simulink model "simplifiedTxTestbench"  (R2024a)
settings: Solver=FixedStepDiscrete  StartTime=0.0  StopTime=stopTime  RelTol=1e-3
values from neighbouring files (symbols this model uses):
  pWords = [pWords binl2str(pBitsRaw)]    [simplifiedTb.m]    (also in tx.m = [pWords binl2str(pBitsRaw{i})])
  reg0 = zeros(length(msgIn), 1)    [tx.m]
  reg1 = zeros(length(msgIn), 1)    [tx.m]
  reg2 = zeros(length(msgIn), 1)    [tx.m]
  reg3 = zeros(length(msgIn), 1)    [tx.m]
undefined symbols (not defined in the file or in its folder): fDAC, fPHY, fs
libraries: dspsrcs4 x3, HDL_ieee_8021513 x2, hdlsllib x1, whdlutilities x1
settings Model: DataTypeOverride=Off  SimulationMode=accelerator  Creator=cotti  LastModifiedBy=cotti
settings OptimizationCC: BlockReduction=off  ConditionallyExecuteInputs=off  DefaultParameterBehavior=Inlined  InheritOutputTypeSmallerThanSingle=on
settings DebuggingCC: ArtificialAlgebraicLoopMsg=error  SingleTaskRateTransMsg=error
settings HardwareCC: ProdBitPerPointer=32  ProdBitPerSizeT=32  ProdBitPerPtrDiffT=32  ProdLargestAtomicFloat=None  ProdIntDivRoundTo=Undefined  ProdEndianess=Unspecified  ProdWordSize=32  ProdHWDeviceType=ASIC/FPGA->ASIC/FPGA  TargetBitPerLong=64  TargetBitPerPointer=64  TargetBitPerSizeT=64  TargetBitPerPtrDiffT=64  TargetLongLongMode=on  TargetIntDivRoundTo=Zero  TargetEndianess=LittleEndian  TargetWordSize=64  TargetHWDeviceType=Custom Processor->MATLAB Host Computer  ProdEqTarget=off

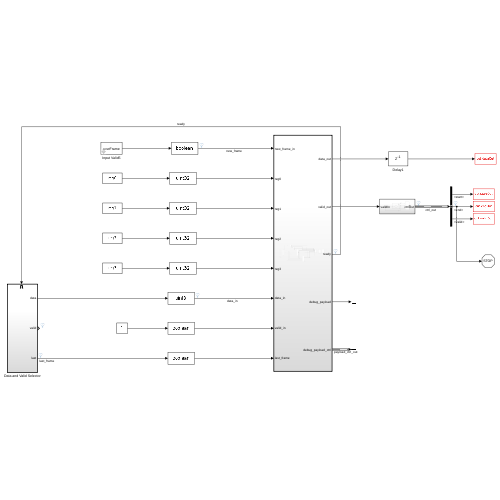
[thumbnail: Simulink's stored preview of the top-level diagram]
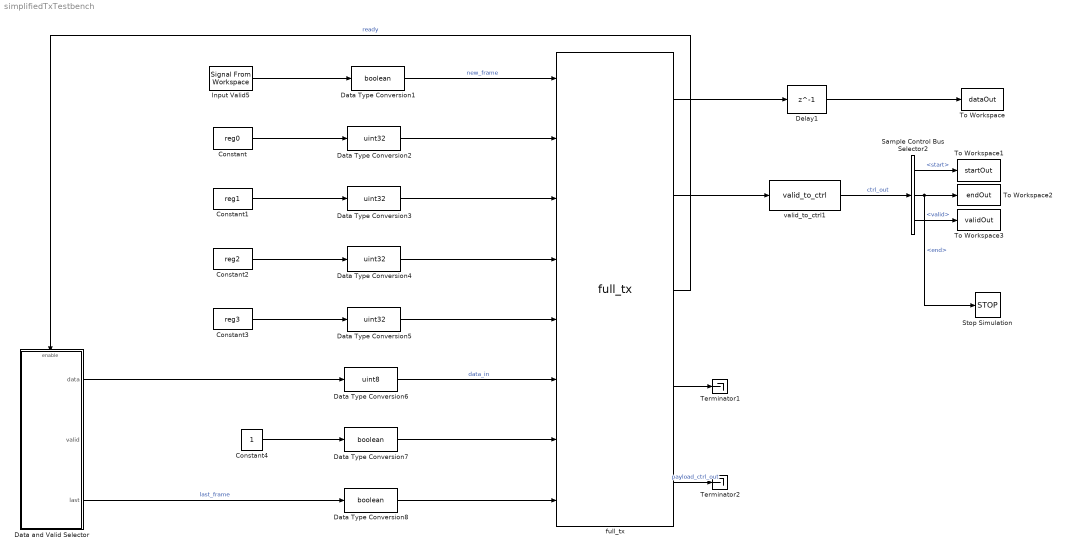
== system simplifiedTxTestbench ==
  Constant : Constant  Value=reg0  OutDataTypeStr=uint32  SampleTime=8/fs
  Constant1 : Constant  Value=reg1  OutDataTypeStr=uint32  SampleTime=8/fs
  Constant2 : Constant  Value=reg2  OutDataTypeStr=uint32  SampleTime=8/fs
  Constant3 : Constant  Value=reg3  OutDataTypeStr=uint32  SampleTime=8/fs
  Constant4 : Constant  SampleTime=-1
  Data Type Conversion1 : DataTypeConversion  OutDataTypeStr=boolean  SaturateOnIntegerOverflow=off  RndMeth=Floor
  Data Type Conversion{2..5} (4 alike) : DataTypeConversion  OutDataTypeStr=uint32  SaturateOnIntegerOverflow=off  RndMeth=Floor
  Data Type Conversion6 : DataTypeConversion  OutDataTypeStr=uint8  SaturateOnIntegerOverflow=off  RndMeth=Floor
  Data Type Conversion7 : DataTypeConversion  OutDataTypeStr=boolean  SaturateOnIntegerOverflow=off  RndMeth=Floor
  Data Type Conversion8 : DataTypeConversion  OutDataTypeStr=boolean  SaturateOnIntegerOverflow=off  RndMeth=Floor
  Data and Valid Selector : Subsystem  TreatAsAtomicUnit=on
  Delay1 : Delay  DelayLength=1  InitialCondition=0  UseCircularBuffer=on
  Input Valid5 : dspsrcs4/Signal From Workspace  X=newFrame  Ts=1/(fPHY/4)  nsamps=1  OutputAfterFinalValue=Setting to zero  ignoreOrWarnInputAndFrameLengths=off  OutputFrames=off
  Sample Control Bus Selector2 : whdlutilities/Sample Control Bus Selector  OutputSignals=start,end,valid
  Stop Simulation : Stop
  Terminator1 : Terminator
  Terminator2 : Terminator
  To Workspace : ToWorkspace  VariableName=dataOut  SampleTime=1/fDAC
      settings: Save2DSignal=2-D array (concatenate along first dimension)
  To Workspace1 : ToWorkspace  VariableName=startOut  SampleTime=1/fDAC
      settings: Save2DSignal=2-D array (concatenate along first dimension)
  To Workspace2 : ToWorkspace  VariableName=endOut  SampleTime=1/fDAC
      settings: Save2DSignal=2-D array (concatenate along first dimension)
  To Workspace3 : ToWorkspace  VariableName=validOut  SampleTime=1/fDAC
      settings: Save2DSignal=2-D array (concatenate along first dimension)
  full_tx : HDL_ieee_8021513/full_tx  SystemSampleTime=-1  VariantActivationTime=update diagram  AllowFlexibleInterface=on  Latency=0  AutoFrameSizeCalculation=off
      settings: SourceProductName=HDL IEEE 8021513
  valid_to_ctrl1 : HDL_ieee_8021513/valid_to_ctrl  SystemSampleTime=-1  VariantActivationTime=update diagram  AllowFlexibleInterface=on  Latency=0  AutoFrameSizeCalculation=off
      settings: SourceProductName=HDL IEEE 8021513
  wires:
  full_tx/3 -> Data and Valid Selector/Enable  "ready"
  Data Type Conversion1/1 -> full_tx/1  "new_frame"
  Data Type Conversion4/1 -> full_tx/4
  Constant2/1 -> Data Type Conversion4/1
  valid_to_ctrl1/1 -> Sample Control Bus Selector2/1  "ctrl_out"
  Data and Valid Selector/1(data) -> Data Type Conversion6/1
  Constant/1 -> Data Type Conversion2/1
  Data Type Conversion5/1 -> full_tx/5
  full_tx/2 -> valid_to_ctrl1/1
  Data and Valid Selector/3(last) -> Data Type Conversion8/1  "last_frame"
  full_tx/1 -> Delay1/1
  Data Type Conversion3/1 -> full_tx/3
  Delay1/1 -> To Workspace/1
  Constant1/1 -> Data Type Conversion3/1
  Sample Control Bus Selector2/3 -> To Workspace3/1  "<valid>"
  Constant3/1 -> Data Type Conversion5/1
  Input Valid5/1 -> Data Type Conversion1/1
  Data Type Conversion2/1 -> full_tx/2
  Sample Control Bus Selector2/1 -> To Workspace1/1  "<start>"
  Data Type Conversion6/1 -> full_tx/6  "data_in"
  Sample Control Bus Selector2/2 -> To Workspace2/1, Stop Simulation/1  "<end>"
  Data Type Conversion8/1 -> full_tx/8
  full_tx/4 -> Terminator1/1
  full_tx/5 -> Terminator2/1  "payload_ctrl_out"
  Constant4/1 -> Data Type Conversion7/1
  Data Type Conversion7/1 -> full_tx/7

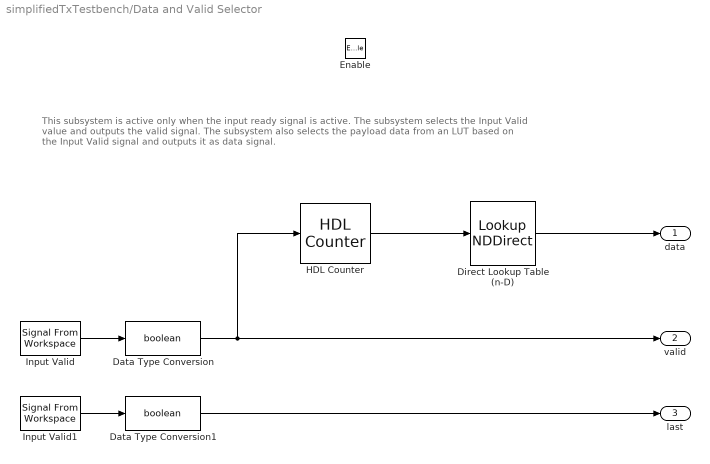
== system simplifiedTxTestbench/Data and Valid Selector ==
  note: This subsystem is active only when the input ready signal is active. The subsystem selects the Input Valid value and outputs the valid signal.
      | The subsystem also selects the payload data from an LUT based on the Input Valid signal and outputs it as data signal.
  Enable : EnablePort
  Data Type Conversion : DataTypeConversion  OutDataTypeStr=boolean  SaturateOnIntegerOverflow=off  RndMeth=Floor
  Data Type Conversion1 : DataTypeConversion  OutDataTypeStr=boolean  SaturateOnIntegerOverflow=off  RndMeth=Floor
  Direct Lookup Table (n-D) : LookupNDDirect  NumberOfTableDimensions=1  Table=uint8(pWords')  DiagnosticForOutOfRangeInput=Error  TableDataTypeStr=uint8
  HDL Counter : hdlsllib/Sources/HDL Counter  CountType=Count limited  CountInit=0  CountStep=1  CountMax=length(pWords) -1  CountFromType=Initial value  CountFrom=0  CountResetPort=off  CountLoadPort=off  CountEnbPort=on  CountDirPort=off  CountHitOutputPort=off  CountDataType=Unsigned  CountWordLen=nextpow2(length(pWords))  CountFracLen=0  CountSampTime=1
  Input Valid : dspsrcs4/Signal From Workspace  X=validIn  Ts=1/(fPHY/4)  nsamps=1  OutputAfterFinalValue=Setting to zero  ignoreOrWarnInputAndFrameLengths=off  OutputFrames=off
  Input Valid1 : dspsrcs4/Signal From Workspace  X=lastIn  Ts=1/(fPHY/4)  nsamps=1  OutputAfterFinalValue=Setting to zero  ignoreOrWarnInputAndFrameLengths=off  OutputFrames=off
  data : Outport  InitialOutput=0  VectorParamsAs1DForOutWhenUnconnected=off
  valid : Outport  Port=2  InitialOutput=0  VectorParamsAs1DForOutWhenUnconnected=off
  last : Outport  Port=3  VectorParamsAs1DForOutWhenUnconnected=off
  wires:
  HDL Counter/1 -> Direct Lookup Table (n-D)/1
  Direct Lookup Table (n-D)/1 -> data/1
  Input Valid/1 -> Data Type Conversion/1
  Data Type Conversion/1 -> valid/1, HDL Counter/1
  Input Valid1/1 -> Data Type Conversion1/1
  Data Type Conversion1/1 -> last/1
